simulink model "nestloop_flex_x2_tb1"  (R2019b)
settings: Solver=VariableStepAuto  StartTime=0.0  StopTime=400  RelTol=1e-3  EnableMultiTasking=on
libraries: simulink x1, lib_dsphdlcontrol_v1 x1
settings Model: Creator=mbabst  LastModifiedBy=mbabst
settings DataIOCC: ReturnWorkspaceOutputs=off
settings OptimizationCC: LifeSpan=inf
settings DebuggingCC: SFUnexpectedBacktrackingDiag=warning  SFNoUnconditionalDefaultTransitionDiag=warning  ArithmeticOperatorsInVariantConditions=warning
settings SFSimCC: SimUseLocalCustomCode=off  CustomCodeUndefinedFunction=UseInterfaceOnly
settings RTWCC: RTWUseLocalCustomCode=off
settings CodeAppCC: StateflowObjectComments=on
settings GRTTargetCC: TargetLangStandard=C89/C90 (ANSI)
settings ConfigComp: CovMetricSettings=dw  CovHtmlReporting=on  CovSaveCumulativeToWorkspaceVar=on  CovSaveSingleToWorkspaceVar=on  CovExternalEMLEnable=off

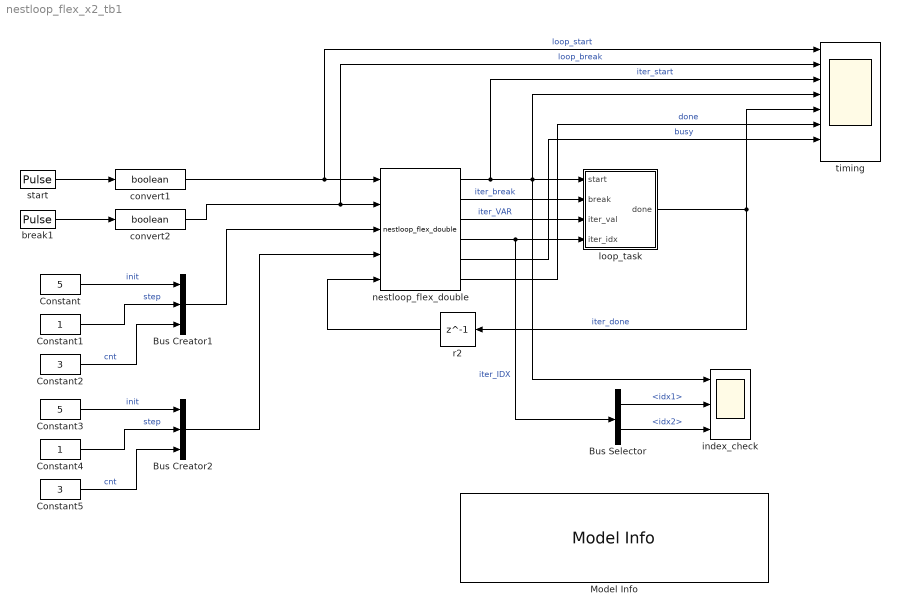
== system nestloop_flex_x2_tb1 ==
  Bus Creator1 : BusCreator  Inputs=3
  Bus Creator2 : BusCreator  Inputs=3
  Bus Selector : BusSelector  OutputSignals=idx1,idx2
  Constant : Constant  Value=5  OutDataTypeStr=fixdt(1,8,4)  SampleTime=1
  Constant1 : Constant  OutDataTypeStr=fixdt(1,8,4)  SampleTime=1
  Constant2 : Constant  Value=3  OutDataTypeStr=fixdt(0,3,0)  SampleTime=1
  Constant3 : Constant  Value=5  OutDataTypeStr=fixdt(1,8,4)  SampleTime=1
  Constant4 : Constant  OutDataTypeStr=fixdt(1,8,4)  SampleTime=1
  Constant5 : Constant  Value=3  OutDataTypeStr=fixdt(0,3,0)  SampleTime=1
  Model Info : simulink/Model-Wide Utilities/Model Info  Frame=on  DisplayStringWithTags=|  HorizontalTextAlignment=Left  LeftAlignmentValue=0.02
      | Copyright (c) 2005-2021 DSPlogic, Inc.
      | Distributed under the terms of the Simplified BSD License.
      | The full license is in the file LICENSE, distributed with this software.
      | 
      | Model: %<ModelName> (v%<ModelVersion>)
      | Author: Michael Babst <mike.babst@dsplogic.com>
      | Created: by %<Creator> on %<Created>
      | Modified: by %<ModifiedBy> on %<LastModificationDate>
  break1 : DiscretePulseGenerator  Period=200  PhaseDelay=130
  convert1 : DataTypeConversion  OutDataTypeStr=boolean
  convert2 : DataTypeConversion  OutDataTypeStr=boolean
  index_check : Scope  NumInputPorts=3
  loop_task : Subsystem
  nestloop_flex_double : lib_dsphdlcontrol_v1/nestloop_flex_double
      settings: SourceProductName=DSPHDL Library
  r2 : Delay  DelayLength=1  InitialCondition=0
  start : DiscretePulseGenerator  Period=100  PhaseDelay=5
  timing : Scope  NumInputPorts=8
  wires:
  start/1 -> convert1/1
  loop_task/1(done) -> timing/5, r2/1  "iter_done"
  convert1/1 -> nestloop_flex_double/1, timing/1  "loop_start"
  Bus Creator1/1 -> nestloop_flex_double/3
  Constant/1 -> Bus Creator1/1  "init"
  Constant1/1 -> Bus Creator1/2  "step"
  Constant2/1 -> Bus Creator1/3  "cnt"
  Bus Creator2/1 -> nestloop_flex_double/4
  Constant3/1 -> Bus Creator2/1  "init"
  Constant4/1 -> Bus Creator2/2  "step"
  Constant5/1 -> Bus Creator2/3  "cnt"
  nestloop_flex_double/1 -> timing/3, timing/4, index_check/1, loop_task/1(start)  "iter_start"
  nestloop_flex_double/3 -> loop_task/3(iter_val)  "iter_VAR"
  nestloop_flex_double/4 -> loop_task/4(iter_idx), Bus Selector/1  "iter_IDX"
  r2/1 -> nestloop_flex_double/5
  nestloop_flex_double/6 -> timing/6  "done"
  nestloop_flex_double/5 -> timing/7  "busy"
  Bus Selector/1 -> index_check/2  "<idx1>"
  Bus Selector/2 -> index_check/3  "<idx2>"
  nestloop_flex_double/2 -> loop_task/2(break)  "iter_break"
  break1/1 -> convert2/1
  convert2/1 -> timing/2, nestloop_flex_double/2  "loop_break"

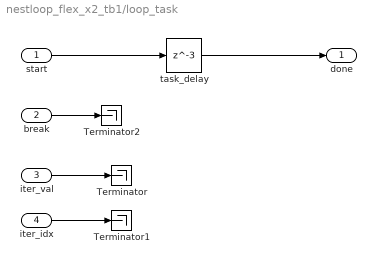
== system nestloop_flex_x2_tb1/loop_task ==
  start : Inport
  break : Inport  Port=2
  iter_val : Inport  Port=3
  iter_idx : Inport  Port=4
  Terminator : Terminator
  Terminator1 : Terminator
  Terminator2 : Terminator
  task_delay : Delay  DelayLength=3  InitialCondition=0
  done : Outport
  wires:
  task_delay/1 -> done/1
  start/1 -> task_delay/1
  iter_val/1 -> Terminator/1
  iter_idx/1 -> Terminator1/1
  break/1 -> Terminator2/1
